simulink model "CC_CV_Adrian_vrs_Emilio"  (R2019a)
settings: Solver=ode23s  StartTime=0.0  StopTime=200  FixedStep=50e-6  RelTol=1e-5
undefined symbols (not defined in the file or in its folder): physconst
libraries: powerlib x16, simulink x9
settings Model: Creator=Soto Porras  LastModifiedBy=juanj
settings DataIOCC: ReturnWorkspaceOutputs=off
settings DebuggingCC: ArithmeticOperatorsInVariantConditions=warning

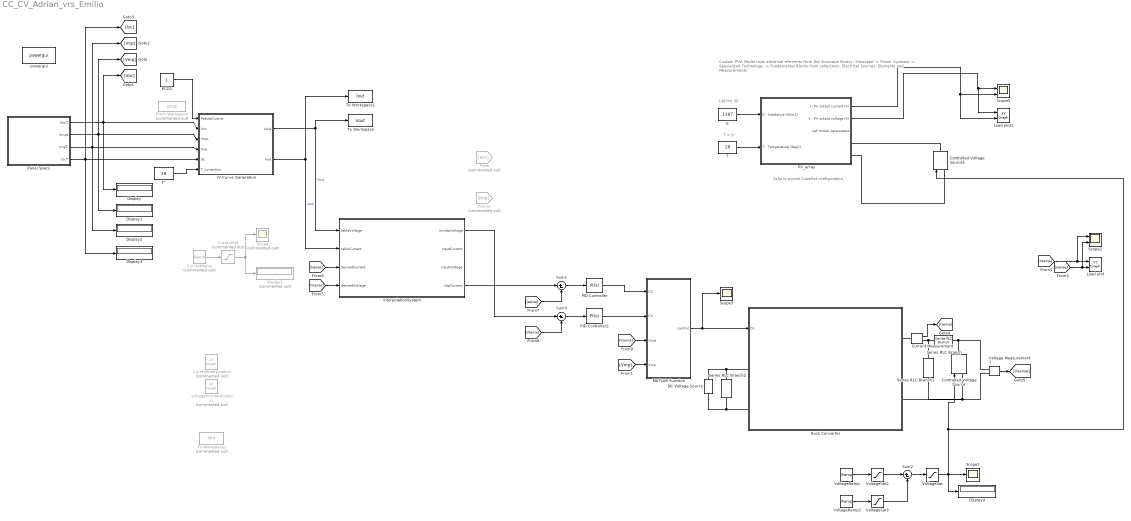
== system CC_CV_Adrian_vrs_Emilio ==
  note: T = 9
  note: Custom PVA
      | Model uses electrical elements from the Simscape library:
      | Simscape -> Power Systems -> Specialized Technology -> Fundamental Blocks
      | from collections: Electrical Sources, Elements and Measurements
  note: 1367*0.35
  note: 2s3p is typical CubeSat configuration
  Buck Converter : Subsystem
  Controlled Voltage Source : powerlib/Electrical Sources/Controlled Voltage Source  Initialize=on  Source_Type=DC  Amplitude=0.1  Phase=0  Frequency=0  Measurements=None
      settings: SourceProductName=Simscape Electrical
  Controlled Voltage Source1 : powerlib/Electrical Sources/Controlled Voltage Source  Initialize=off  Source_Type=DC  Amplitude=0  Phase=0  Frequency=0  Measurements=None
  Current Measurement : powerlib/Measurements/Current Measurement  PhasorSimulation=off  OutputType=Complex  PSBequivalent=0
      settings: SourceProductName=Simscape Electrical
  CurrentInterpolation : simulink/Sinks/XY Graph  Commented=on  xmin=0  xmax=6  ymin=0  ymax=2  st=-1
  CurrentRamp : simulink/Sources/Ramp  Commented=on  slope=0.015603  start=0  InitialOutput=0
  CurrentSat : Saturate  Commented=on  UpperLimit=1.5603  LowerLimit=0
  DC Voltage Source : powerlib/Electrical Sources/DC Voltage Source  Amplitude=15  Measurements=None
      settings: SourceProductName=Simscape Electrical
  Display{,1..4} (5 alike) : Display
  Display5 : Display  Commented=on
  E : Constant  Value=1367
  From : From  Commented=on  GotoTag=Voc
  From Workspace : FromWorkspace  Commented=on  VariableName=pcos  SampleTime=0
  From2 : From  Commented=on  GotoTag=Imp
  IV Curve Generation : Subsystem  mask(Panel I-V Curve Calculation){ValueVocComp=0.0062, ValueVmpComp=0.0067}
      mask prompts: ValueVocComp "Voc Temperature Correction (V)"; ValueVmpComp "Vmp Temperature Correction (V)"
      mask help:
      | This module calculates the panel IV curve using the next panel parameters:
      | 1. Voc
      | 2. Vmp
      | 3. Imp
      | 4. Isc
      |
      | It applies:
      | 1. Correction to current parameters (Isc and Imp) using a pseudo cosine that varies depending on the angle of the perpendicular CubeSat face and the sun's incident radiation.
      | 2. Correction to voltage parameters (Voc and Vmp) using the panel datasheet voltage losses, given in V by the user.
      mask TypeOptions ValueVocComp: Voc_comp/Value
      mask TypeOptions ValueVmpComp: Vmp_comp/Value
      mask Display: image('IV_curve.png');
  InterpolationSystem : Subsystem
  Load plot : simulink/Sinks/XY Graph  xmin=0  xmax=6  ymin=0  ymax=2  st=-1
  Load plot1 : simulink/Sinks/XY Graph  xmin=0  xmax=6  ymin=0  ymax=2  st=-1
  MATLAB Function : MATLAB Function  TreatAsAtomicUnit=on
  PCOS : Constant
  PID Controller : simulink/Continuous/PID Controller  Controller=PI  Form=Parallel  TimeDomain=Continuous-time  SampleTime=0.00005  IntegratorMethod=Trapezoidal  FilterMethod=Forward Euler  ControllerParametersSource=internal  P=10  I=0.01  D=0  UseFilter=on  N=100  TunerSelectOption=Frequency Response Based  InitialConditionSource=internal  InitialConditionForIntegrator=0  InitialConditionForFilter=0  DifferentiatorICPrevScaledInput=0  ExternalReset=none  TrackingMode=off  Kt=1  LimitOutput=off  UpperSaturationLimit=0.9  LowerSaturationLimit=0.1  LinearizeAsGain=on  AntiWindupMode=none  Kb=1  POutMin=[]  POutMax=[]  IOutMin=[]  IOutMax=[]  DOutMin=[]  DOutMax=[]  NOutMin=[]  NOutMax=[]  SumOutMin=[]  SumOutMax=[]  SaturationOutMin=[]  SaturationOutMax=[]  PParamMin=[]  PParamMax=[]  IParamMin=[]  IParamMax=[]  DParamMin=[]  DParamMax=[]  NParamMin=[]  NParamMax=[]  KbParamMin=[]  KbParamMax=[]  KtParamMin=[]  KtParamMax=[]  KbOutMin=[]  KbOutMax=[]  KtOutMin=[]  KtOutMax=[]  IntegratorOutMin=[]  IntegratorOutMax=[]  FilterOutMin=[]  FilterOutMax=[]  SumI1OutMin=[]  SumI1OutMax=[]  SumI2OutMin=[]  SumI2OutMax=[]  SumI3OutMin=[]  SumI3OutMax=[]  SumI4OutMin=[]  SumI4OutMax=[]  SumDOutMin=[]  SumDOutMax=[]  DifferentiatorOutMin=[]  DifferentiatorOutMax=[]  FilterDiffOutCoefMin=[]  FilterDiffOutCoefMax=[]  ReciprocalOutMin=[]  ReciprocalOutMax=[]  SumDenOutMin=[]  SumDenOutMax=[]  SumNumOutMin=[]  SumNumOutMax=[]  DivideOutMin=[]  DivideOutMax=[]  IntegratorContinuousStateAttributes=''  IntegratorStateMustResolveToSignalObject=off  IntegratorRTWStateStorageClass=Auto  FilterContinuousStateAttributes=''  FilterStateMustResolveToSignalObject=off  FilterRTWStateStorageClass=Auto  ParallelPVariant=InternalParameters  IdealPVariant=Disabled  IVariant=InternalParameters  DVariant=Disabled  IntegratorVariant=Continuous  SatVariant=Disabled  AWVariant=Passthrough  PCopyVariant=Disabled  TRVariant=Disabled  FdbkBlocksVariant=Forward  IdealPFdbkVariant=Disabled  SatFdbkVariant=Disabled  DerivativeFilterVariant=Disabled  NVariant=Disabled  NCopyVariant=Disabled_SignalSpec  FilterICVariant=Disabled  IntegratorICVariant=InternalICs  ExternalResetVariant=Disabled  TRSumVariant=Passthrough  SumFdbkVariant=Disabled  SumVariant=Sum_PI
  PID Controller2 : simulink/Continuous/PID Controller  Controller=PI  Form=Parallel  TimeDomain=Continuous-time  SampleTime=0.00005  IntegratorMethod=Trapezoidal  FilterMethod=Forward Euler  ControllerParametersSource=internal  P=10  I=0.0001  D=0.01  UseFilter=on  N=100  TunerSelectOption=Transfer Function Based (PID Tuner App)  InitialConditionSource=internal  InitialConditionForIntegrator=0  InitialConditionForFilter=0  DifferentiatorICPrevScaledInput=0  ExternalReset=none  TrackingMode=off  Kt=1  LimitOutput=off  UpperSaturationLimit=0.9  LowerSaturationLimit=0.1  LinearizeAsGain=on  AntiWindupMode=none  Kb=1  POutMin=[]  POutMax=[]  IOutMin=[]  IOutMax=[]  DOutMin=[]  DOutMax=[]  NOutMin=[]  NOutMax=[]  SumOutMin=[]  SumOutMax=[]  SaturationOutMin=[]  SaturationOutMax=[]  PParamMin=[]  PParamMax=[]  IParamMin=[]  IParamMax=[]  DParamMin=[]  DParamMax=[]  NParamMin=[]  NParamMax=[]  KbParamMin=[]  KbParamMax=[]  KtParamMin=[]  KtParamMax=[]  KbOutMin=[]  KbOutMax=[]  KtOutMin=[]  KtOutMax=[]  IntegratorOutMin=[]  IntegratorOutMax=[]  FilterOutMin=[]  FilterOutMax=[]  SumI1OutMin=[]  SumI1OutMax=[]  SumI2OutMin=[]  SumI2OutMax=[]  SumI3OutMin=[]  SumI3OutMax=[]  SumI4OutMin=[]  SumI4OutMax=[]  SumDOutMin=[]  SumDOutMax=[]  DifferentiatorOutMin=[]  DifferentiatorOutMax=[]  FilterDiffOutCoefMin=[]  FilterDiffOutCoefMax=[]  ReciprocalOutMin=[]  ReciprocalOutMax=[]  SumDenOutMin=[]  SumDenOutMax=[]  SumNumOutMin=[]  SumNumOutMax=[]  DivideOutMin=[]  DivideOutMax=[]  IntegratorContinuousStateAttributes=''  IntegratorStateMustResolveToSignalObject=off  IntegratorRTWStateStorageClass=Auto  FilterContinuousStateAttributes=''  FilterStateMustResolveToSignalObject=off  FilterRTWStateStorageClass=Auto  ParallelPVariant=InternalParameters  IdealPVariant=Disabled  IVariant=InternalParameters  DVariant=Disabled  IntegratorVariant=Continuous  SatVariant=Disabled  AWVariant=Passthrough  PCopyVariant=Disabled  TRVariant=Disabled  FdbkBlocksVariant=Forward  IdealPFdbkVariant=Disabled  SatFdbkVariant=Disabled  DerivativeFilterVariant=Disabled  NVariant=Disabled  NCopyVariant=Disabled_SignalSpec  FilterICVariant=Disabled  IntegratorICVariant=InternalICs  ExternalResetVariant=Disabled  TRSumVariant=Passthrough  SumFdbkVariant=Disabled  SumVariant=Sum_PI
  PV_array : Subsystem  mask(PV Array Model){s=2, p=3, n=2.5, T_ref=28, E_ref=1367, Voc_ref=2690, Isc_ref=519.6, Vmp_ref=2409, Imp_ref=502.9, kVoc=-6.2, kIsc=0.36, kVmp=-6.7, kImp=0.24}
      mask prompts: s "Serial cells (s)"; p "Parallel cells (p)"; n "Diode ideality factor / emission coefficient (n)"; T_ref "Temperature (degC), T_ref"; E_ref "Irradiation (W/m2), E_ref"; Voc_ref "Open circuit voltage (mV), Voc"; Isc_ref "Short circuit current (mA), Isc"; Vmp_ref "Voltage @ mpp (mV), Vmp"; Imp_ref "Current @ mpp (mA), Imp"; kVoc "Delta Voc / Delta T (mV/degC), kVoc"; kIsc "Delta Isc / Delta T (mA/degC), kIsc"; kVmp "Delta Vmp / Delta T (mV/degC), kVmp"; kImp "Delta Imp / Delta T (mA/degC), kImp"
      mask help:
      | This block models a PVA through the single diode solar cell model, scaled by the number of serial (s) and parallel (p) cells.
      | The diode ideality factor (n) of the model must be chosen. Reasonable values for n are 1.5 ... 2.5.
      | - Input: irradiance, cell temperature
      | - Output: electrical connections (current/voltage)
      mask init:
      | %% Input parameters for determination of 'Rs' initial guess
      | T_in = 0;      % [deg C] - Temperature (typical cell temperature)
      | 
      | %% Constants
      | k = 1.38064852e-23;          % [J/K] - Boltzmann constant
      | q = 1.6021766208e-19;        % [As]  - Elementary charge
      | 
      | %% Calculations
      | % Temperature dependent quantities
      | Vt = 1000*k*(T_in+273.15)/q;   % [mV] - thermal voltage
      | Isc = Isc_ref + (T_in - T_ref) * kIsc;
      | Voc = Voc_ref + (T_in - T_ref) * kVoc;
      | Imp = Imp_ref + (T_in - T_ref) * kImp;
      | Vmp = Vmp_ref + (T_in - T_ref) * kVmp;
      | % Determining Rs
      | n_diode = n;
      | syms Rs_sym
      | Term1 = simplify((n_diode*Vt*Vmp*(2*Imp-Isc))/((Vmp*Isc+Voc*(Imp-Isc))*(Vmp-Imp*Rs_sym)-n_diode*Vt*(Vmp*Isc-Voc*Imp)), 'Steps', 100);
      | Term2 = simplify(exp((Vmp+Imp*Rs_sym-Voc)/(n_diode*Vt)), 'Steps', 100);
      | Rs_sym = solve(Term1==Term2, Rs_sym);
      | Rs = double(Rs_sym);
      | 
      | % Set Rs as initial guess in solver block
      | set_param([gcb '/get_5_model_parameters/get_Rs/solve_Rs'], 'z0', num2str(Rs));
      mask Help:
      | - Input: irradiance, cell temperature
      | - Output: electrical connections (current/voltage)
      | 
      | - Single diode solar cell model
      | - Setup: current source, parallel diode, shunt and series resistor
      | - Block parameters are the solar cell data sheet values
      | - Model determines the 5 parameters of the single diode solar cell model (Iph, Isat, n, Rsh, Rs, where n must be chosen) using the block inputs and the block parameters, based on the approach of Villalva et al., 2009
      | - The 5 calculated model parameters are used to control an internal parametrized current source
      | - Model parameters are determined using Voc, Isc, V and I @ MPP and the corresponding temperature dependencies of the modeled solar cell as given in the data sheet
      | 
      | - n: Diode ideality factor (1.5...2.5 for reasonable results)
      | 
      | - CAUTION: when choosing a higher ideality factor (n) and/or when applying extreme temperatures, the modeled shunt resistance may result in a negative value. This is not critical, as the model does not claim to correspond to reality, only to depict it. However, this can be prevented by reducing (n).
      mask TypeOptions s: serial_cells/Value
      mask TypeOptions p: parallel_cells/Value
      mask TypeOptions n: get_5_model_parameters/n
      mask TypeOptions T_ref: get_5_model_parameters/T_ref
      mask TypeOptions E_ref: get_5_model_parameters/E_ref
      mask TypeOptions Voc_ref: get_5_model_parameters/Voc_ref
      mask TypeOptions Isc_ref: get_5_model_parameters/Isc_ref
      mask TypeOptions Vmp_ref: get_5_model_parameters/Vmp_ref
      mask TypeOptions Imp_ref: get_5_model_parameters/Imp_ref
      mask TypeOptions kVoc: get_5_model_parameters/kVoc
      mask TypeOptions kIsc: get_5_model_parameters/kIsc
      mask TypeOptions kVmp: get_5_model_parameters/kVmp
      mask TypeOptions kImp: get_5_model_parameters/kImp
      mask DialogControl Container5 Prompt: PV Array Configuration
      mask DialogControl Container9 Prompt: Model Parameterization
      mask DialogControl n Tooltip: Choose a valuue from 1.5 ... 2.5 for reasonable results
      mask DialogControl Container7 Prompt: Cell Parameters (as given in the data sheet)
      mask DialogControl ParameterGroupVar Prompt: Conditions of reference measurement
      mask DialogControl Container3 Prompt: Characteristics (reference measurement @ T_ref, E_ref)
      mask DialogControl Container4 Prompt: Temperature coefficients
  Panel Specs : Subsystem  mask(Solar Panel Specifications){Voc=2.690, Vmp=2.409, Imp=0.5029, Isc=0.5196, SerialGain=2, ParallelGain=3}
      mask prompts: SerialGain "Serial"; ParallelGain "Parallel"
      mask help: Inputs solar panel electrical specifications, temperature and array distribution.
      mask TypeOptions Voc: Voc/Value
      mask TypeOptions Vmp: Vmp/Value
      mask TypeOptions Imp: Imp/Value
      mask TypeOptions Isc: Isc/Value
      mask TypeOptions SerialGain: Gain/Gain | Gain1/Gain
      mask TypeOptions ParallelGain: Gain2/Gain | Gain3/Gain
      mask DialogControl Container3 Prompt: Panel Array
      mask Display: image('solar_panel.png');
  Scope : Scope  Commented=on
  Scope1 : Scope
  Scope2 : Scope  NumInputPorts=2
  Scope3 : Scope
  Scope5 : Scope  NumInputPorts=2
  Series RLC Branch : powerlib/Elements/Series RLC Branch  LConnTagsString=__new0  RConnTagsString=__new0  BranchType=R  Resistance=1e-3  Inductance=1e-3  SetiL0=off  InitialCurrent=0  Capacitance=1e-6  Setx0=off  InitialVoltage=0  Measurements=None
      settings: SourceProductName=Simscape Electrical
  Series RLC Branch1 : powerlib/Elements/Series RLC Branch  LConnTagsString=__new0  RConnTagsString=__new0  BranchType=RC  Resistance=1e-2  Inductance=1e-3  SetiL0=off  InitialCurrent=0  Capacitance=100e-6  Setx0=off  InitialVoltage=0  Measurements=None
      settings: SourceProductName=Simscape Electrical
  Series RLC Branch2 : powerlib/Elements/Series RLC Branch  LConnTagsString=__new0  RConnTagsString=__new0  BranchType=RC  Resistance=1e-3  Inductance=1e-3  SetiL0=off  InitialCurrent=0  Capacitance=100e-6  Setx0=off  InitialVoltage=0  Measurements=None
      settings: SourceProductName=Simscape Electrical
  Sum1 : Sum  Inputs=|+-
  Sum2 : Sum  Inputs=|+-
  Sum3 : Sum  Inputs=|+-
  T : Constant  Value=28
  To Workspace : ToWorkspace  VariableName=Vout  SaveFormat=Structure With Time  SampleTime=-1
  To Workspace1 : ToWorkspace  VariableName=Iout  SaveFormat=Structure With Time  SampleTime=-1
  To Workspace2 : ToWorkspace  Commented=on  VariableName=Vint  SaveFormat=Structure With Time  SampleTime=-1
  T° : Constant  Value=28
  Voltage Measurement1 : powerlib/Measurements/Voltage Measurement  PhasorSimulation=off  OutputType=Complex  PSBequivalent=0
      settings: SourceProductName=Simscape Electrical
  VoltageInvInterpolation : simulink/Sinks/XY Graph  Commented=on  xmin=0  xmax=6  ymin=0  ymax=2  st=-1
  VoltageRamp : simulink/Sources/Ramp  slope=0.0538  start=0  InitialOutput=0
  VoltageRamp2 : simulink/Sources/Ramp  slope=0.0538  start=100  InitialOutput=0
  VoltageSat : Saturate  UpperLimit=5.2  LowerLimit=0.1
  VoltageSat2 : Saturate  UpperLimit=5.35  LowerLimit=0.1
  VoltageSat3 : Saturate  UpperLimit=5.35  LowerLimit=0.1
  powergui : powerlib/powergui  Priority=1  SimulationMode=Continuous  SampleTime=50e-6  frequency=60  Iterations=50  frequencyindice=0  Pbase=100e6  ErrMax=1e-4  UnitsV=kV  UnitsW=MW  buscounter=0  FunctionMessages=off  echomessages=off  EnableUseOfTLC=off  CurrentSourceSwitches=off  DisableSnubberDevices=off  DisableRonSwitches=off  DisableVfSwitches=off  DisplayEquations=off  AutomaticDiscreteSolvers=off  SolverType=Tustin/Backward Euler (TBE)  Interpol=off  ExternalGateDelay=off  methode=off  Ts=100  x0status=blocks  SPID=on  SwTol=0  HookPort=off  NonlinearTolerance=0  nMaxIteration=15  ContinueOnMaxIteration=off  RestoreLinks=warning  ResistiveCurrentMeasurement=off  Frange=[0:2:500]  Ylog=off  Xlog=on  ShowGrid=off  save=off  variable=ZData  structure=0  ZoomFFT=off  StartTime=0.0  cycles=1  DisplayStyle=1  fundamental=60  FreqAxis=off  MaxFrequency=1000  frequencyindicesteady=1  RmsSteady=1  display=off
      settings: SourceProductName=Simscape Electrical
  wires:
  Panel Specs/1(VocT) -> [Voc], Display/1, IV Curve Generation/2(Voc)
  Panel Specs/2(Vmpt) -> [Vmp], Display1/1, IV Curve Generation/3(Vmp)
  Panel Specs/3(ImpT) -> [Imp], Display2/1, IV Curve Generation/4(Imp)
  Panel Specs/4(IscT) -> [Isc], Display3/1, IV Curve Generation/5(Isc)
  CurrentRamp/1 -> CurrentSat/1
  IV Curve Generation/1(Vout) -> InterpolationSystem/1(tableVoltage), To Workspace/1  "Vout"
  IV Curve Generation/2(Iout) -> To Workspace1/1, InterpolationSystem/2(tableCurrent)  "Iout"
  CurrentSat/1 -> Display5/1, Scope/1
  T°/1 -> IV Curve Generation/6(T_correction)
  Sum1/1 -> PID Controller/1
  VoltageSat/1 -> Controlled Voltage Source1/1, Controlled Voltage Source/1, Scope1/1, Display4/1
  Voltage Measurement1/1 -> [Vsense]
  Current Measurement/1 -> [Isense]
  InterpolationSystem/4(intpCurrent) -> Sum1/1
  PID Controller/1 -> MATLAB Function/1(CC)
  MATLAB Function/1(control) -> Scope3/1, Buck Converter/1(Dc)
  PID Controller2/1 -> MATLAB Function/2(CV)
  Sum3/1 -> PID Controller2/1
  InterpolationSystem/1(invIntpVoltage) -> Sum3/1
  [Isense] -> Scope2/2, Load plot/2
  [Vsense] -> Scope2/1, Load plot/1
  [Vsense] -> InterpolationSystem/4(desiredVotlage)
  [Isense] -> InterpolationSystem/3(desiredCurrent)
  [Isense] -> Sum1/2
  [Vsense] -> Sum3/2
  [Vsense] -> MATLAB Function/3(Vout)
  [Vmp] -> MATLAB Function/4(Vmp)
  PCOS/1 -> IV Curve Generation/1(PseudoCosine)
  Sum2/1 -> VoltageSat/1
  VoltageRamp/1 -> VoltageSat2/1
  VoltageSat2/1 -> Sum2/1
  VoltageRamp2/1 -> VoltageSat3/1
  VoltageSat3/1 -> Sum2/2
  PV_array/1(I - PV output current (A)) -> Scope5/2, Load plot1/2
  T/1 -> PV_array/2(T - Temperature (degC))
  PV_array/2(V - PV output voltage (V)) -> Load plot1/1, Scope5/1
  E/1 -> PV_array/1(E - Irradiance (W/m2))
  connections:
  DC Voltage Source/RConn1 -- Series RLC Branch2/LConn1 -- Buck Converter/LConn1
  DC Voltage Source/LConn1 -- Series RLC Branch2/RConn1 -- Buck Converter/LConn2
  Voltage Measurement1/LConn2 -- Series RLC Branch1/RConn1 -- Buck Converter/RConn2 -- Controlled Voltage Source/LConn1
  Series RLC Branch/LConn1 -- Controlled Voltage Source/RConn1 -- Voltage Measurement1/LConn1
  Current Measurement/LConn1 -- Buck Converter/RConn1
  Current Measurement/RConn1 -- Series RLC Branch1/LConn1 -- Series RLC Branch/RConn1
  Controlled Voltage Source1/RConn1 -- PV_array/RConn1
  Controlled Voltage Source1/LConn1 -- PV_array/RConn2

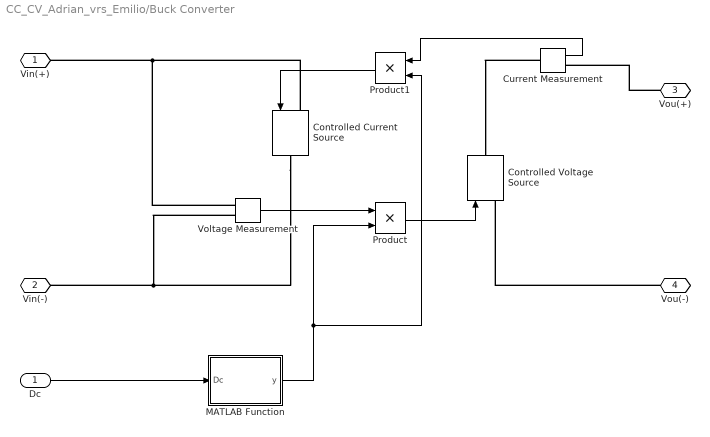
== system CC_CV_Adrian_vrs_Emilio/Buck Converter ==
  Dc : Inport
  Controlled Current Source : powerlib/Electrical Sources/Controlled Current Source  Initialize=off  Source_Type=DC  Amplitude=0  Phase=0  Frequency=0  Measurements=None
      settings: SourceProductName=Simscape Electrical
  Controlled Voltage Source : powerlib/Electrical Sources/Controlled Voltage Source  Initialize=off  Source_Type=DC  Amplitude=0  Phase=0  Frequency=0  Measurements=None
      settings: SourceProductName=Simscape Electrical
  Current Measurement : powerlib/Measurements/Current Measurement  PhasorSimulation=off  OutputType=Complex  PSBequivalent=0
      settings: SourceProductName=Simscape Electrical
  MATLAB Function : MATLAB Function  TreatAsAtomicUnit=on
  Product : Product
  Product1 : Product
  Voltage Measurement : powerlib/Measurements/Voltage Measurement  PhasorSimulation=off  OutputType=Complex  PSBequivalent=0
      settings: SourceProductName=Simscape Electrical
  Vin(+) : PMIOPort  Side=Left
  Vin(-) : PMIOPort  Port=2  Side=Left
  Vou(+) : PMIOPort  Port=3  Side=Right
  Vou(-) : PMIOPort  Port=4  Side=Right
  wires:
  Product/1 -> Controlled Voltage Source/1
  Current Measurement/1 -> Product1/1
  Product1/1 -> Controlled Current Source/1
  MATLAB Function/1(y) -> Product1/2, Product/2
  Voltage Measurement/1 -> Product/1
  Dc/1 -> MATLAB Function/1(Dc)
  connections:
  Controlled Current Source/RConn1 -- Voltage Measurement/LConn2 -- Vin(-)/RConn1
  Vou(-)/RConn1 -- Controlled Voltage Source/LConn1
  Current Measurement/LConn1 -- Controlled Voltage Source/RConn1
  Controlled Current Source/LConn1 -- Voltage Measurement/LConn1 -- Vin(+)/RConn1
  Vou(+)/RConn1 -- Current Measurement/RConn1

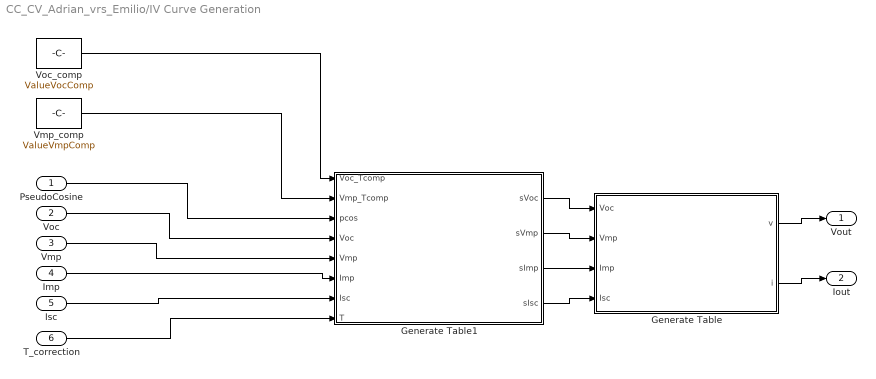
== system CC_CV_Adrian_vrs_Emilio/IV Curve Generation ==
  PseudoCosine : Inport
  Voc : Inport  Port=2
  Vmp : Inport  Port=3
  Imp : Inport  Port=4
  Isc : Inport  Port=5
  T_correction : Inport  Port=6
  Generate Table : MATLAB Function  TreatAsAtomicUnit=on
  Generate Table1 : MATLAB Function  TreatAsAtomicUnit=on
  Vmp_comp : Constant  Value=ValueVmpComp
  Voc_comp : Constant  Value=ValueVocComp
  Vout : Outport
  Iout : Outport  Port=2
  wires:
  Isc/1 -> Generate Table1/7(Isc)
  Generate Table1/4(sIsc) -> Generate Table/4(Isc)
  Voc_comp/1 -> Generate Table1/1(Voc_Tcomp)
  Generate Table/1(v) -> Vout/1
  T_correction/1 -> Generate Table1/8(T)
  Generate Table1/2(sVmp) -> Generate Table/2(Vmp)
  Voc/1 -> Generate Table1/4(Voc)
  Generate Table1/3(sImp) -> Generate Table/3(Imp)
  Imp/1 -> Generate Table1/6(Imp)
  Generate Table1/1(sVoc) -> Generate Table/1(Voc)
  Vmp/1 -> Generate Table1/5(Vmp)
  Generate Table/2(i) -> Iout/1
  Vmp_comp/1 -> Generate Table1/2(Vmp_Tcomp)
  PseudoCosine/1 -> Generate Table1/3(pcos)

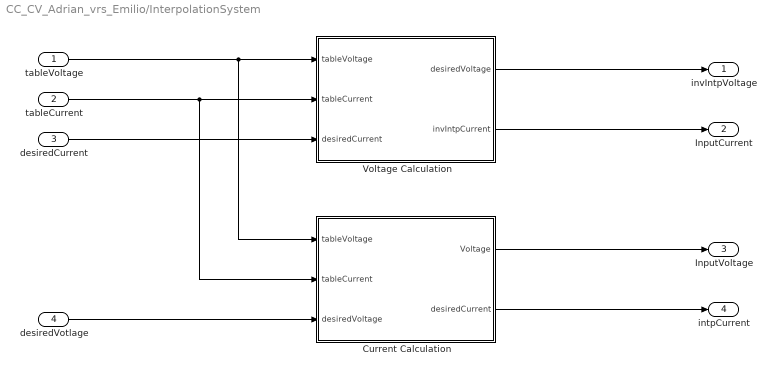
== system CC_CV_Adrian_vrs_Emilio/InterpolationSystem ==
  tableVoltage : Inport
  tableCurrent : Inport  Port=2
  desiredCurrent : Inport  Port=3
  desiredVotlage : Inport  Port=4
  Current Calculation : MATLAB Function  TreatAsAtomicUnit=on
  Voltage Calculation : MATLAB Function  TreatAsAtomicUnit=on
  invIntpVoltage : Outport
  InputCurrent : Outport  Port=2
  InputVoltage : Outport  Port=3
  intpCurrent : Outport  Port=4
  wires:
  Current Calculation/1(Voltage) -> InputVoltage/1
  Voltage Calculation/1(desiredVoltage) -> invIntpVoltage/1
  tableVoltage/1 -> Voltage Calculation/1(tableVoltage), Current Calculation/1(tableVoltage)
  Current Calculation/2(desiredCurrent) -> intpCurrent/1
  tableCurrent/1 -> Voltage Calculation/2(tableCurrent), Current Calculation/2(tableCurrent)
  Voltage Calculation/2(invIntpCurrent) -> InputCurrent/1
  desiredCurrent/1 -> Voltage Calculation/3(desiredCurrent)
  desiredVotlage/1 -> Current Calculation/3(desiredVoltage)

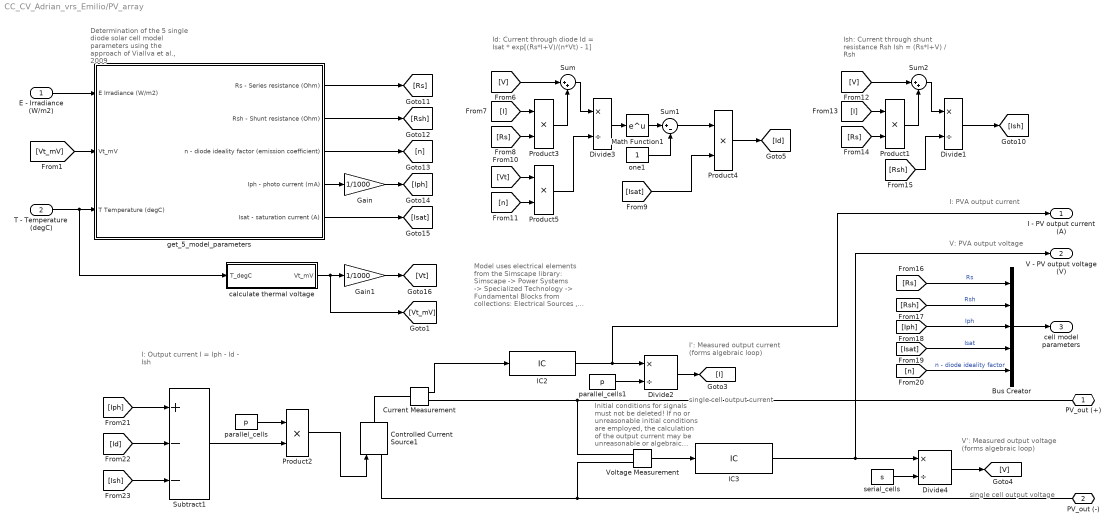
== system CC_CV_Adrian_vrs_Emilio/PV_array ==
  note: single cell output current
  note: single cell output voltage
  note: Determination of the 5 single diode solar cell model parameters
      | using the approach of Viallva et al., 2009
  note: Id: Current through diode
      |
      | Id = Isat * exp[(Rs*I+V)/(n*Vt) - 1]
  note: Ish: Current through shunt resistance Rsh
      |
      | Ish = (Rs*I+V) / Rsh
  note: I': Measured output current
      | (forms algebraic loop)
  note: I: Output current
      |
      | I = Iph - Id - Ish
  note: V': Measured output voltage
      | (forms algebraic loop)
  note: Initial conditions for signals must not be deleted!
      | If no or unreasonable initial conditions are employed, the calculation of the
      | output current may be unreasonable or algebraic loops may not be solved.
  note: Model uses electrical elements from the Simscape library:
      | Simscape -> Power Systems -> Specialized Technology -> Fundamental Blocks
      | from collections: Electrical Sources , Elements and Measurements
  note: I: PVA output current
  note: V: PVA output voltage
  E - Irradiance (W/m2) : Inport
  T - Temperature (degC) : Inport  Port=2
  Bus Creator : BusCreator  Inputs=5
  Controlled Current Source1 : powerlib/Electrical Sources/Controlled Current Source  Initialize=on  Source_Type=DC  Amplitude=0  Phase=0  Frequency=0  Measurements=None
  Current Measurement : powerlib/Measurements/Current Measurement  PhasorSimulation=off  OutputType=Complex  PSBequivalent=0
  Divide{1..4} (4 alike) : Product  Inputs=*/
  Gain : Gain  Gain=1/1000
  Gain1 : Gain  Gain=1/1000
  IC2 : InitialCondition  Value=(Imp_ref*p)/1000
  IC3 : InitialCondition  Value=(Vmp_ref*s)/1000/2
  Math Function1 : Math  SaturateOnIntegerOverflow=on
  Product{1..5} (5 alike) : Product
  Subtract1 : Sum  Inputs=+--
  Sum : Sum  Inputs=|++
  Sum1 : Sum  Inputs=|+-
  Sum2 : Sum  Inputs=|++
  Voltage Measurement : powerlib/Measurements/Voltage Measurement  PhasorSimulation=off  OutputType=Complex  PSBequivalent=0
  calculate thermal voltage : Subsystem
  get_5_model_parameters : Subsystem  mask(Parameter identifier of "single diode" solar cell model){n=n, T_ref=T_ref, E_ref=E_ref, Voc_ref=Voc_ref, Isc_ref=Isc_ref, Vmp_ref=Vmp_ref, Imp_ref=Imp_ref, kVoc=kVoc, kIsc=kIsc, kVmp=kVmp, kImp=kImp}
      mask prompts: n "Diode ideality factor (emission coefficient)"; T_ref "Temperature (degC), T_ref ="; E_ref "Irradiation (W/m2), E_ref ="; Voc_ref "Open circuit voltage (mV), Voc"; Isc_ref "Short circuit current (mA), Isc"; Vmp_ref "Voltage @ mpp (mV), Vmp"; Imp_ref "Current @ mpp (mA), Imp"; kVoc "Delta Voc / Delta T (mV/degC), kVoc"; kIsc "Delta Isc / Delta T (mA/degC), kIsc"; kVmp "Delta Vmp / Delta T (mV/degC), kVmp"; kImp "Delta Imp / Delta T (mA/degC), kImp"
      mask help:
      | - solar cell model, type: single diode + innert losses
      | - using a current source, parallel diode, shunt and series resistor
      | - output: 5 parameters (Iph, Isat, n, Rsh, Rs)
      | - input: irradiance, temperature
      | - model parameters aret determined using Voc, Isc, V and I @ mpp and the corresponding temperature coefficients
      mask DialogControl Container5 Prompt: Tunable model parameters
      mask DialogControl n Tooltip: Choose a valuue from 1.5 ... 2.5 for reasonable results
      mask DialogControl ParameterGroupVar Prompt: Conditions of reference measurement
      mask DialogControl Container8 Prompt: Characteristics (reference measurement @ T_ref, E_ref)
      mask DialogControl Container9 Prompt: Temperature dependencies
  one1 : Constant
  parallel_cells : Constant  Value=p
  parallel_cells1 : Constant  Value=p
  serial_cells : Constant  Value=s
  PV_out (+) : PMIOPort  Side=Right
  PV_out (-) : PMIOPort  Port=2  Side=Right
  I - PV output current (A) : Outport
  V - PV output voltage (V) : Outport  Port=2
  cell model parameters : Outport  Port=3
  wires:
  Gain/1 -> [Iph]
  [I] -> Product1/1
  Product1/1 -> Sum2/2
  [V] -> Sum2/1
  Divide3/1 -> Math Function1/1
  one1/1 -> Sum1/2
  Sum/1 -> Divide3/1
  [V] -> Sum/1
  Sum1/1 -> Product4/1
  [Rs] -> Product1/2
  Product3/1 -> Sum/2
  Math Function1/1 -> Sum1/1
  [Isat] -> Product4/2
  [Rsh] -> Divide1/2
  Product4/1 -> [Id]
  [Vt] -> Product5/1
  [n] -> Product5/2
  [I] -> Product3/1
  Product5/1 -> Divide3/2
  calculate thermal voltage/1(Vt_mV) -> [Vt_mV], Gain1/1
  get_5_model_parameters/4(Iph - photo current (mA)) -> Gain/1
  get_5_model_parameters/1(Rs - Series resistance (Ohm)) -> [Rs]
  get_5_model_parameters/5(Isat - saturation current (A)) -> [Isat]
  Sum2/1 -> Divide1/1
  Divide1/1 -> [Ish]
  get_5_model_parameters/2(Rsh - Shunt resistance (Ohm)) -> [Rsh]
  Gain1/1 -> [Vt]
  [Rs] -> Product3/2
  E - Irradiance (W/m2)/1 -> get_5_model_parameters/1(E Irradiance (W/m2))
  get_5_model_parameters/3(n - diode ideality factor (emission coefficient)) -> [n]
  IC3/1 -> Divide4/1, V - PV output voltage (V)/1
  [Rs] -> Bus Creator/1  "Rs"
  [Rsh] -> Bus Creator/2  "Rsh"
  [Iph] -> Bus Creator/3  "Iph"
  [Isat] -> Bus Creator/4  "Isat"
  Bus Creator/1 -> cell model parameters/1
  [n] -> Bus Creator/5  "n - diode ideality factor"
  Current Measurement/1 -> IC2/1
  [Ish] -> Subtract1/3
  [Id] -> Subtract1/2
  Voltage Measurement/1 -> IC3/1
  Subtract1/1 -> Product2/2
  parallel_cells/1 -> Product2/1
  Divide2/1 -> [I]
  Divide4/1 -> [V]
  Product2/1 -> Controlled Current Source1/1
  IC2/1 -> I - PV output current (A)/1, Divide2/1
  parallel_cells1/1 -> Divide2/2
  serial_cells/1 -> Divide4/2
  T - Temperature (degC)/1 -> get_5_model_parameters/3(T Temperature (degC)), calculate thermal voltage/1(T_degC)
  [Vt_mV] -> get_5_model_parameters/2(Vt_mV)
  [Iph] -> Subtract1/1
  connections:
  Controlled Current Source1/RConn1 -- Current Measurement/LConn1
  PV_out (-)/RConn1 -- Voltage Measurement/LConn2 -- Controlled Current Source1/LConn1
  Voltage Measurement/LConn1 -- PV_out (+)/RConn1 -- Current Measurement/RConn1

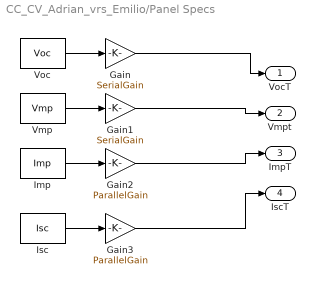
== system CC_CV_Adrian_vrs_Emilio/Panel Specs ==
  Gain : Gain  Gain=SerialGain
  Gain1 : Gain  Gain=SerialGain
  Gain2 : Gain  Gain=ParallelGain
  Gain3 : Gain  Gain=ParallelGain
  Imp : Constant  Value=Imp
  Isc : Constant  Value=Isc
  Vmp : Constant  Value=Vmp
  Voc : Constant  Value=Voc
  VocT : Outport
  Vmpt : Outport  Port=2
  ImpT : Outport  Port=3
  IscT : Outport  Port=4
  wires:
  Isc/1 -> Gain3/1
  Vmp/1 -> Gain1/1
  Gain/1 -> VocT/1
  Imp/1 -> Gain2/1
  Gain2/1 -> ImpT/1
  Gain3/1 -> IscT/1
  Voc/1 -> Gain/1
  Gain1/1 -> Vmpt/1

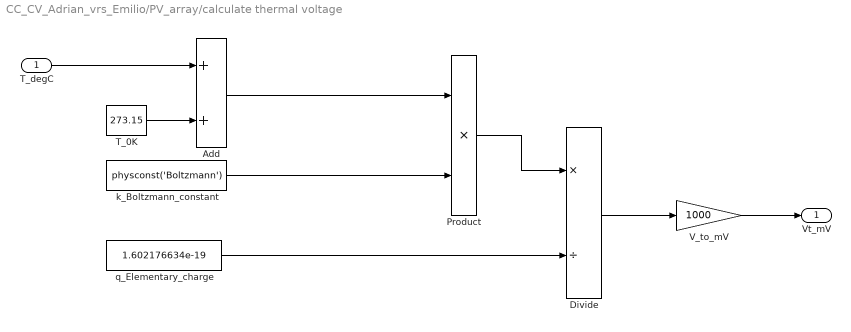
== system CC_CV_Adrian_vrs_Emilio/PV_array/calculate thermal voltage ==
  T_degC : Inport
  Add : Sum
  Divide : Product  Inputs=*/
  Product : Product
  T_0K : Constant  Value=273.15
  V_to_mV : Gain  Gain=1000
  k_Boltzmann_constant : Constant  Value=physconst('Boltzmann')
  q_Elementary_charge : Constant  Value=1.602176634e-19
  Vt_mV : Outport
  wires:
  Product/1 -> Divide/1
  Divide/1 -> V_to_mV/1
  k_Boltzmann_constant/1 -> Product/2
  V_to_mV/1 -> Vt_mV/1
  q_Elementary_charge/1 -> Divide/2
  Add/1 -> Product/1
  T_degC/1 -> Add/1
  T_0K/1 -> Add/2

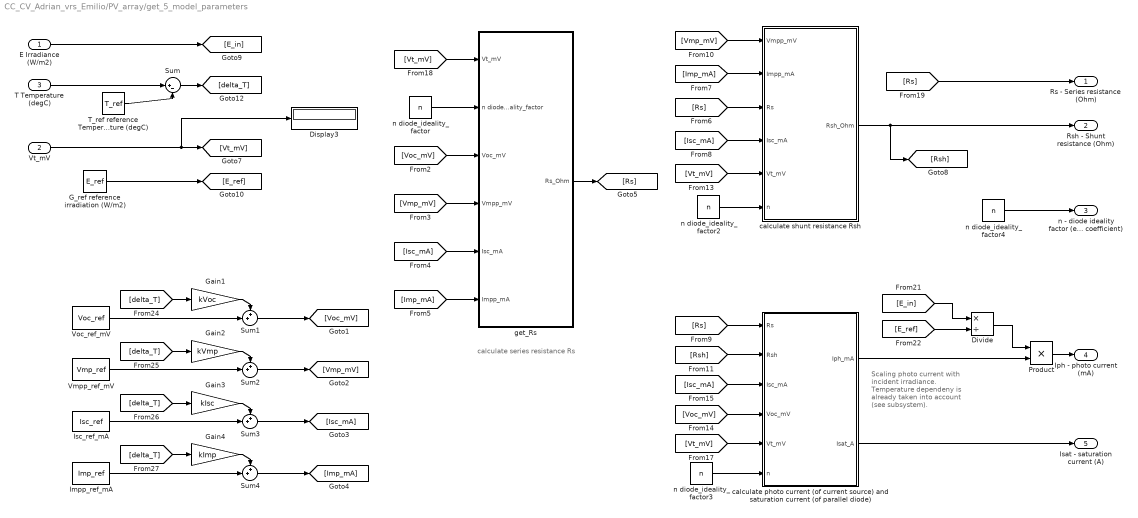
== system CC_CV_Adrian_vrs_Emilio/PV_array/get_5_model_parameters ==
  note: calculate series resistance Rs
  note: Scaling photo current with incident irradiance.
      | Temperature dependeny is already taken into
      | account (see subsystem).
  E Irradiance (W/m2) : Inport
  Vt_mV : Inport  Port=2
  T Temperature (degC) : Inport  Port=3
  Display3 : Display
  Divide : Product  Inputs=*/
  G_ref reference irradiation (W/m2) : Constant  Value=E_ref
  Gain1 : Gain  Gain=kVoc
  Gain2 : Gain  Gain=kVmp
  Gain3 : Gain  Gain=kIsc
  Gain4 : Gain  Gain=kImp
  Impp_ref_mA : Constant  Value=Imp_ref
  Isc_ref_mA : Constant  Value=Isc_ref
  Product : Product
  Sum : Sum  Inputs=|+-
  Sum{1..4} (4 alike) : Sum  Inputs=++|
  T_ref reference Temperature (degC) : Constant  Value=T_ref
  Vmpp_ref_mV : Constant  Value=Vmp_ref
  Voc_ref_mV : Constant  Value=Voc_ref
  calculate photo current (of current source) and saturation current (of parallel diode) : Subsystem
  calculate shunt resistance Rsh : Subsystem
  get_Rs : Subsystem
  n diode_ideality_factor{,2..4} (4 alike) : Constant  Value=n
  Rs - Series resistance (Ohm) : Outport
  Rsh - Shunt resistance (Ohm) : Outport  Port=2
  n - diode ideality factor (emission coefficient) : Outport  Port=3
  Iph - photo current (mA) : Outport  Port=4
  Isat - saturation current (A) : Outport  Port=5
  wires:
  [Vt_mV] -> get_Rs/1(Vt_mV)
  [Imp_mA] -> get_Rs/6(Impp_mA)
  [Vmp_mV] -> get_Rs/4(Vmpp_mV)
  [Isc_mA] -> get_Rs/5(Isc_mA)
  [Voc_mV] -> get_Rs/3(Voc_mV)
  get_Rs/1(Rs_Ohm) -> [Rs]
  [Rs] -> calculate photo current (of current source) and saturation current (of parallel diode)/1(Rs)
  calculate photo current (of current source) and saturation current (of parallel diode)/2(Isat_A) -> Isat - saturation current (A)/1
  [Voc_mV] -> calculate photo current (of current source) and saturation current (of parallel diode)/4(Voc_mV)
  [Imp_mA] -> calculate shunt resistance Rsh/2(Impp_mA)
  [Vt_mV] -> calculate shunt resistance Rsh/5(Vt_mV)
  [Vt_mV] -> calculate photo current (of current source) and saturation current (of parallel diode)/5(Vt_mV)
  [Rs] -> calculate shunt resistance Rsh/3(Rs)
  [Isc_mA] -> calculate shunt resistance Rsh/4(Isc_mA)
  [Vmp_mV] -> calculate shunt resistance Rsh/1(Vmpp_mV)
  [Isc_mA] -> calculate photo current (of current source) and saturation current (of parallel diode)/3(Isc_mA)
  [Rsh] -> calculate photo current (of current source) and saturation current (of parallel diode)/2(Rsh)
  calculate shunt resistance Rsh/1(Rsh_Ohm) -> Rsh - Shunt resistance (Ohm)/1, [Rsh]
  T Temperature (degC)/1 -> Sum/1
  [Rs] -> Rs - Series resistance (Ohm)/1
  E Irradiance (W/m2)/1 -> [E_in]
  [E_in] -> Divide/1
  Product/1 -> Iph - photo current (mA)/1
  G_ref reference irradiation (W/m2)/1 -> [E_ref]
  [E_ref] -> Divide/2
  T_ref reference Temperature (degC)/1 -> Sum/2
  Sum/1 -> [delta_T]
  [delta_T] -> Gain1/1
  Voc_ref_mV/1 -> Sum1/2
  Gain1/1 -> Sum1/1
  Gain2/1 -> Sum2/1
  Vmpp_ref_mV/1 -> Sum2/2
  [delta_T] -> Gain2/1
  [delta_T] -> Gain4/1
  Impp_ref_mA/1 -> Sum4/2
  Gain4/1 -> Sum4/1
  Gain3/1 -> Sum3/1
  Isc_ref_mA/1 -> Sum3/2
  [delta_T] -> Gain3/1
  Sum1/1 -> [Voc_mV]
  Sum2/1 -> [Vmp_mV]
  Sum3/1 -> [Isc_mA]
  Sum4/1 -> [Imp_mA]
  Vt_mV/1 -> Display3/1, [Vt_mV]
  n diode_ideality_factor2/1 -> calculate shunt resistance Rsh/6(n)
  n diode_ideality_factor3/1 -> calculate photo current (of current source) and saturation current (of parallel diode)/6(n)
  n diode_ideality_factor4/1 -> n - diode ideality factor (emission coefficient)/1
  calculate photo current (of current source) and saturation current (of parallel diode)/1(Iph_mA) -> Product/2
  Divide/1 -> Product/1
  n diode_ideality_factor/1 -> get_Rs/2(n diode_ideality_factor)

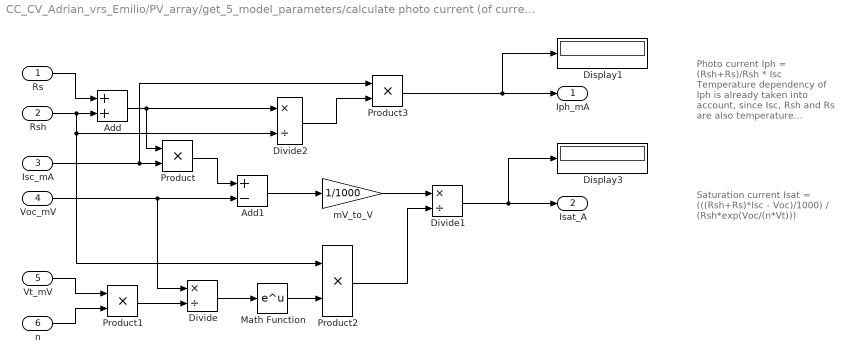
== system CC_CV_Adrian_vrs_Emilio/PV_array/get_5_model_parameters/calculate photo current (of current source) and saturation current (of parallel diode) ==
  note: Saturation current
      | Isat = (((Rsh+Rs)*Isc - Voc)/1000) / (Rsh*exp(Voc/(n*Vt)))
  note: Photo current
      | Iph = (Rsh+Rs)/Rsh * Isc
      |
      | Temperature dependency of Iph is already taken into account,
      | since Isc, Rsh and Rs are also temperature dependent.
  Rs : Inport
  Rsh : Inport  Port=2
  Isc_mA : Inport  Port=3
  Voc_mV : Inport  Port=4
  Vt_mV : Inport  Port=5
  n : Inport  Port=6
  Add : Sum
  Add1 : Sum  Inputs=+-
  Display1 : Display
  Display3 : Display
  Divide : Product  Inputs=*/
  Divide1 : Product  Inputs=*/
  Divide2 : Product  Inputs=*/
  Math Function : Math  SaturateOnIntegerOverflow=on
  Product{,1..3} (4 alike) : Product
  mV_to_V : Gain  Gain=1/1000
  Iph_mA : Outport
  Isat_A : Outport  Port=2
  wires:
  Product2/1 -> Divide1/2
  Isc_mA/1 -> Product3/1, Product/2
  Divide/1 -> Math Function/1
  Voc_mV/1 -> Add1/2, Divide/1
  Product1/1 -> Divide/2
  Vt_mV/1 -> Product1/1
  Rs/1 -> Add/1
  Add1/1 -> mV_to_V/1
  n/1 -> Product1/2
  Divide1/1 -> Display3/1, Isat_A/1
  Product/1 -> Add1/1
  Rsh/1 -> Divide2/2, Product2/1, Add/2
  mV_to_V/1 -> Divide1/1
  Add/1 -> Product/1, Divide2/1
  Math Function/1 -> Product2/2
  Divide2/1 -> Product3/2
  Product3/1 -> Display1/1, Iph_mA/1

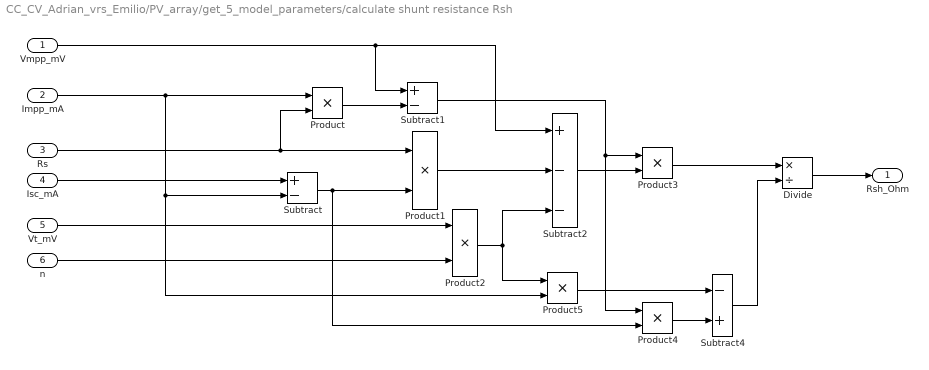
== system CC_CV_Adrian_vrs_Emilio/PV_array/get_5_model_parameters/calculate shunt resistance Rsh ==
  Vmpp_mV : Inport
  Impp_mA : Inport  Port=2
  Rs : Inport  Port=3
  Isc_mA : Inport  Port=4
  Vt_mV : Inport  Port=5
  n : Inport  Port=6
  Divide : Product  Inputs=*/
  Product{,1..5} (6 alike) : Product
  Subtract : Sum  Inputs=+-
  Subtract1 : Sum  Inputs=+-
  Subtract2 : Sum  Inputs=+--
  Subtract4 : Sum  Inputs=-+
  Rsh_Ohm : Outport
  wires:
  Subtract4/1 -> Divide/2
  Product3/1 -> Divide/1
  Product5/1 -> Subtract4/1
  Rs/1 -> Product/2, Product1/1
  Isc_mA/1 -> Subtract/1
  Product1/1 -> Subtract2/2
  Vmpp_mV/1 -> Subtract1/1, Subtract2/1
  n/1 -> Product2/2
  Vt_mV/1 -> Product2/1
  Subtract1/1 -> Product4/1, Product3/1
  Divide/1 -> Rsh_Ohm/1
  Product2/1 -> Subtract2/3, Product5/1
  Subtract/1 -> Product1/2, Product4/2
  Product/1 -> Subtract1/2
  Subtract2/1 -> Product3/2
  Product4/1 -> Subtract4/2
  Impp_mA/1 -> Subtract/2, Product5/2, Product/1

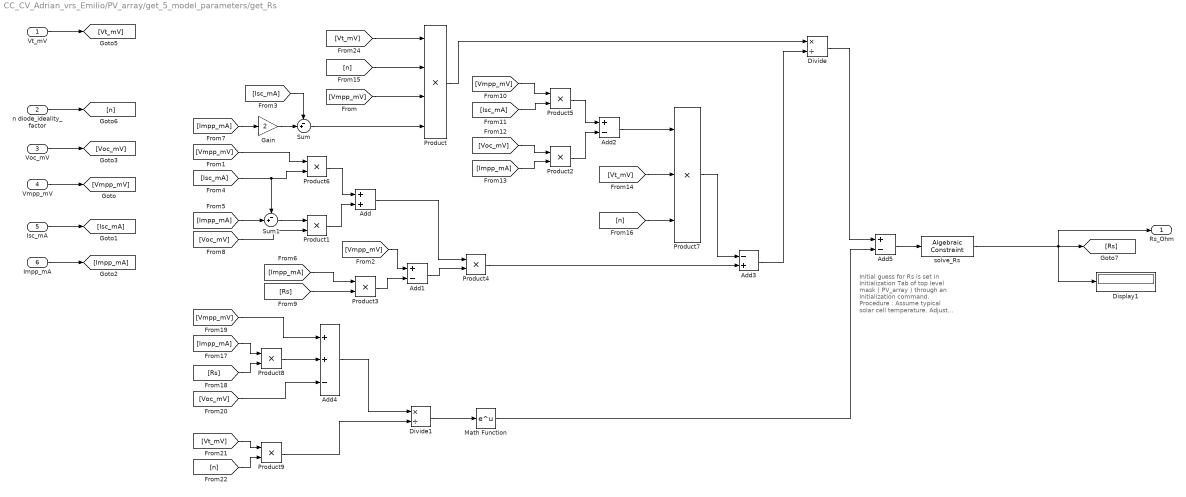
== system CC_CV_Adrian_vrs_Emilio/PV_array/get_5_model_parameters/get_Rs ==
  note: Initial guess for Rs is set in Initialization Tab of top level mask
      | ( PV_array ) through an Initialization command.
      |
      | Procedure :
      | Assume typical solar cell temperature.
      | Adjust Voc, Isc, Vmp, Imp according to their temperature
      | coefficients and the solar cell temperature.
      | Determine Rs for chosen n value (diode emission factor set
      | through top level mask) using the approach of Villalva et al., 2009
      | with the Equations and systems solver from Matlab.
      | Set found Rs as initial guess parameter in the Simulink Algebraic
      | Constraints Block that solves for Rs during simulation.
  Vt_mV : Inport
  n diode_ideality_factor : Inport  Port=2
  Voc_mV : Inport  Port=3
  Vmpp_mV : Inport  Port=4
  Isc_mA : Inport  Port=5
  Impp_mA : Inport  Port=6
  Add : Sum
  Add1 : Sum  Inputs=+-
  Add2 : Sum  Inputs=+-
  Add3 : Sum  Inputs=-+
  Add4 : Sum  Inputs=++-
  Add5 : Sum  Inputs=+-
  Display1 : Display
  Divide : Product  Inputs=*/
  Divide1 : Product  Inputs=*/
  Gain : Gain  Gain=2
  Math Function : Math  SaturateOnIntegerOverflow=on
  Product : Product  Inputs=4
  Product{1..6,8..9} (8 alike) : Product
  Product7 : Product  Inputs=3
  Sum : Sum  Inputs=-+|
  Sum1 : Sum  Inputs=-+|
  solve_Rs : AlgebraicConstraint  InitialGuess=0.087875
  Rs_Ohm : Outport
  wires:
  [Vmpp_mV] -> Add1/1
  Vmpp_mV/1 -> [Vmpp_mV]
  [Voc_mV] -> Add4/3
  Product7/1 -> Add3/1
  [Voc_mV] -> Product1/2
  [Vt_mV] -> Product/1
  [Voc_mV] -> Product2/1
  [Vmpp_mV] -> Add4/1
  Gain/1 -> Sum/2
  Product2/1 -> Add2/2
  [Vmpp_mV] -> Product/3
  Divide/1 -> Add5/1
  Product9/1 -> Divide1/2
  [n] -> Product/2
  [Vt_mV] -> Product7/2
  [Vmpp_mV] -> Product5/1
  [Impp_mA] -> Product8/1
  [Impp_mA] -> Sum1/2
  [Vmpp_mV] -> Product6/1
  Product5/1 -> Add2/1
  [Isc_mA] -> Sum/1
  [Impp_mA] -> Gain/1
  [Rs] -> Product3/2
  [n] -> Product7/3
  [Impp_mA] -> Product3/1
  Add/1 -> Product4/1
  Add2/1 -> Product7/1
  Divide1/1 -> Math Function/1
  n diode_ideality_factor/1 -> [n]
  Product1/1 -> Add/2
  Sum/1 -> Product/4
  [Vt_mV] -> Product9/1
  Add5/1 -> solve_Rs/1
  Add3/1 -> Divide/2
  [Isc_mA] -> Product5/2
  Product6/1 -> Add/1
  Vt_mV/1 -> [Vt_mV]
  Impp_mA/1 -> [Impp_mA]
  Isc_mA/1 -> [Isc_mA]
  Product3/1 -> Add1/2
  Sum1/1 -> Product1/1
  Voc_mV/1 -> [Voc_mV]
  Product8/1 -> Add4/2
  Add1/1 -> Product4/2
  Product/1 -> Divide/1
  [Rs] -> Product8/2
  [n] -> Product9/2
  [Impp_mA] -> Product2/2
  Add4/1 -> Divide1/1
  [Isc_mA] -> Sum1/1, Product6/2
  solve_Rs/1 -> Rs_Ohm/1, [Rs], Display1/1
  Math Function/1 -> Add5/2
  Product4/1 -> Add3/2

== matlab function CC_CV_Adrian_vrs_Emilio/Buck Converter/MATLAB Function ==
  data: Dc input; y output
function y = M(Dc)
y = Dc;

== matlab function CC_CV_Adrian_vrs_Emilio/InterpolationSystem/Voltage Calculation ==
  data: desiredVoltage output; tableVoltage input; tableCurrent input; invIntpCurrent output; desiredCurrent input
function [desiredVoltage, invIntpCurrent] = CurrentInverseInterpolation(tableVoltage, tableCurrent, desiredCurrent)
    
    % Apply inverse interpolation on ampere ramp values
    n = 1024;
    v = 0;
    %i = 1023;
    for j = 1 : n - 1
        i = 1024 - j;
        if(desiredCurrent < tableCurrent(i))
           v = tableVoltage(i) + (tableVoltage(i+1)-tableVoltage(i))*((desiredCurrent - tableCurrent(i))/(tableCurrent(i+1) - tableCurrent(i)));
           break;
        end
    end
     desiredVoltage = v;
     invIntpCurrent = desiredCurrent;
    
end

== matlab function CC_CV_Adrian_vrs_Emilio/IV Curve Generation/Generate Table ==
  data: Voc input; Vmp input; Imp input; Isc input; v output; i output
function [v,i] = generate_table(Voc, Vmp, Imp, Isc)
Rs = ( Voc - Vmp ) / Imp;
a = ( Vmp * ( 1 + ( Rs*Isc ) / Voc ) + Rs*( Imp - Isc ) ) / Voc;
N = log( 2 - 2^a) / log ( Imp / Isc );
i=zeros(1024,1);
v=zeros(1024,1);
for x = 1:1024
    I = (x * Isc) / 1023.0;
    V = Voc * log( 2 - ( ( I / Isc ) ^ N ) );
    V = V / log( 2 );
    V = V - Rs * ( I - Isc );
    V = V / ( 1 + ( ( Rs * Isc) / Voc) );
    P = V * I;
    v(x) = V;
    i(x) = I;
end
v = flip(v);
i = flip(i);

== matlab function CC_CV_Adrian_vrs_Emilio/InterpolationSystem/Current Calculation ==
  data: Voltage output; desiredCurrent output; tableVoltage input; tableCurrent input; desiredVoltage input
function [Voltage, desiredCurrent] = VoltageInterpolation(tableVoltage, tableCurrent, desiredVoltage)
    
    % Apply interpolation on voltage ramp values
    n = 1023;
    c = 0;
    for j = 1 : n + 1
        i = j;
        if(desiredVoltage < tableVoltage(i))
           c = tableCurrent(i) + ...
               (tableCurrent(i-1)-tableCurrent(i))*...
               ((desiredVoltage - tableVoltage(i))/(tableVoltage(i-1) - tableVoltage(i)));
           break;
        end
    end

    
%     for i = 1 : n
%         vi = tableVoltage(i);
%         for j = 1 : n
%             if(j ~= i)
%                 vi = vi*((y-tableCurrent(j))/(tableCurrent(i) - tableCurrent(j)));
%             end
%         end
%         invIntpVoltageHelper = invIntpVoltageHelper + vi;
%     end
% 
     desiredCurrent = c;
     Voltage = desiredVoltage;
    
end

== matlab function CC_CV_Adrian_vrs_Emilio/MATLAB Function ==
  data: CC input; control output; CV input; Vout input; Vmp input
function control = CC_CV(CC,CV,Vout,Vmp)

    if Vout >= Vmp
        control = CV;
    else 
        control = CC;
end

== matlab function CC_CV_Adrian_vrs_Emilio/IV Curve Generation/Generate Table1 ==
  data: Voc_Tcomp input; Vmp_Tcomp input; pcos input; Voc input; Vmp input; Imp input; Isc input; sVoc output; sVmp output; sImp output; sIsc output; T input
function [sVoc, sVmp, sImp, sIsc] = scalevars(Voc_Tcomp, Vmp_Tcomp, pcos, Voc, Vmp, Imp, Isc, T)
sVoc = Voc-(T*Voc_Tcomp);
sVmp = Vmp-(T*Vmp_Tcomp);
sImp = pcos * Imp;
sIsc = pcos * Isc;
